simulink model "A_Simple_Calculator"  (R2018b)
settings: Solver=FixedStepDiscrete  StartTime=0.0  StopTime=10.0  RelTol=1e-3
settings Model: Creator=Peter Ghali  LastModifiedBy=Peter Ghali
settings OptimizationCC: DefaultParameterBehavior=Inlined  EnhancedBackFolding=on  PassReuseOutputArgsAs=Individual arguments  OptimizeBlockOrder=speed  DifferentSizesBufferReuse=on  OptimizationCustomize=off
settings DebuggingCC: ParameterTunabilityLossMsg=error
settings SFSimCC: MATLABDynamicMemAlloc=off
settings RTWCC: SystemTargetFile=ert.tlc  GenCodeOnly=on  TemplateMakefile=ert_default_tmf  GenerateReport=on  IncludeHyperlinkInReport=on  LaunchReport=on  GenerateTraceInfo=on  GenerateTraceReport=on  GenerateTraceReportSl=on  GenerateTraceReportSf=on  GenerateTraceReportEml=on
settings CodeAppCC: ForceParamTrailComments=on  IgnoreCustomStorageClasses=off  OperatorAnnotations=on  SimulinkDataObjDesc=on  SFDataObjDesc=on  InsertBlockDesc=on
settings ERTTargetCC: TargetLangStandard=C99 (ISO)  GenerateSampleERTMain=on  InlinedParameterPlacement=NonHierarchical  ERTCustomFileTemplate=example_file_process.tlc

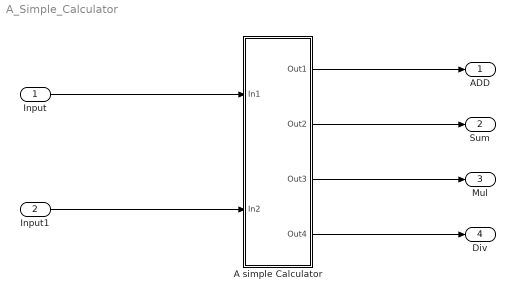
== system A_Simple_Calculator ==
  Input : Inport
  Input1 : Inport  Port=2
  A simple Calculator : Subsystem  TreatAsAtomicUnit=on
  ADD : Outport
  "Sum " : Outport  Port=2
  "Mul " : Outport  Port=3
  "Div " : Outport  Port=4
  wires:
  Input/1 -> A simple Calculator/1(In1)
  Input1/1 -> A simple Calculator/2(In2)
  A simple Calculator/1(Out1) -> ADD/1
  A simple Calculator/2(Out2) -> "Sum "/1
  A simple Calculator/3(Out3) -> "Mul "/1
  A simple Calculator/4(Out4) -> "Div "/1

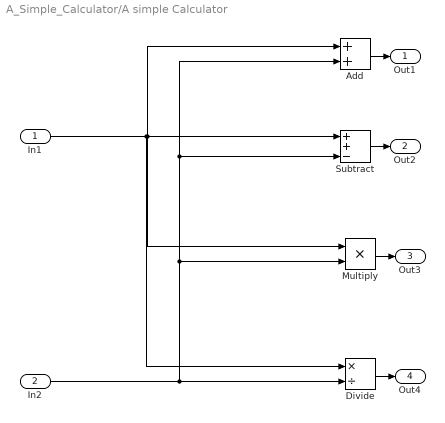
== system A_Simple_Calculator/A simple Calculator ==
  In1 : Inport
  In2 : Inport  Port=2
  Add : Sum
  Divide : Product  Inputs=*/
  Multiply : Product
  Subtract : Sum  Inputs=++-
  Out1 : Outport
  Out2 : Outport  Port=2
  Out3 : Outport  Port=3
  Out4 : Outport  Port=4
  wires:
  In1/1 -> Multiply/1, Subtract/1, Add/1, Divide/1
  Divide/1 -> Out4/1
  Multiply/1 -> Out3/1
  In2/1 -> Add/2, Subtract/3, Multiply/2, Divide/2
  Add/1 -> Out1/1
  Subtract/1 -> Out2/1
